simulink model "NeuronalNetwork"  (R2019b)
settings: Solver=VariableStepAuto  StartTime=0.0  StopTime=10.0  RelTol=1e-3
libraries: neural x1006
(part 4 of 11)

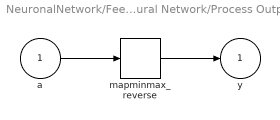
== system NeuronalNetwork/Feed-Forward Neural Network/Process Output 1 ==
  a : Inport  PortDimensions=1001  SampleTime=0.1
      mask Display: e = 0.06;c1 = [120 230 180]/255;c2 = ([120 230 180]+0)/(256+128);c3 = ([120 230 180]+128)/(256+128);patch([0 1 1 0],[0 0 1 1],c1);patch([0 1 1 1-e 1-e 0+e],[0 0 1 1-e 0+e 0+e],c2);patch([0 0 1 1-e 0+e 0+e],[0 1 1 1-e 1-e 0+e],c3);plot([0 1 1 0 0],[0 0 1 1 0]);
  mapminmax_reverse : neural/Processing Functions/mapminmax_reverse  xmin=[1.28539816339744827899949086714;1.20368306698340132854241346649;1.13712353826944823076416923868;1.08663227213241242452568258159;1.04879801985670040309628348041;1.01840689604369138976380781969;0.990200914007079879830541813135;0.959785932234298533316518842184;0.923951810884579005644923199725;0.880690181190778353936821076786;0.82910523056761875615450207988;0.769305868941106085756587162905;0.702287253703623770562103345583;0.629773356468130929286530772515;0.553998001771835668627375071082;0.477432717740583156817990584386;0.402501528649066797616029589335;0.331335469164235618677594175097;0.265607673356772433503891761575;0.206463137107515737334040295536;0.154531156045622314332277369431;0.109993530356310459383806232836;0.0726795004890897489158163580214;0.0421645837339916507158221747886;0.017859386511117698176365209406;-0.0009177424313119231713206658263;-0.0148851418599052279234662421459;-0.0247575410518087804523368333776;-0.0312182369750025681676142141896;-0.0349009375278889616422972608234;-0.0363788753059904115816358682878;-0.0361593048566425795398160403238;-0.034681949339717889346790258287;-0.0323203135455749288040827593704;-0.0293850345279976013501688214546;-0.026128622222722015094875658292;-0.0227510749875170885381248098156;-0.0194059579004072363384025834421;-0.0162066168017704972936776641745;-0.01323227471824351894613691627;-0.0105338220429840728753489997871;-0.00813916833642066434029160859609;-0.00605807183182810026628173361019;-0.00428640265499571643942333665223;-0.00280982765288581310542115332396;-0.00160692915066506809146362755314;-0.000651787741753224840468572409691;8.39286851426477892475219722002e-05;0.000629320082254218463382877679635;0.00101300031231716714842649995632;0.00126218020832500016185917512956;0.00140203514486378095355023631896;0.00145530765965246706647451269134;0.00144209971760712353516797890052;0.00137981388265491153322095385647;0.00128320762461004876306414068665;0.00116452998530110055953878944734;0.00103371466977684837995621336404;0.000898608179116162182273330749638;0.000765215770345728692192199815736;0.000637951762407977778640555399647;0.000519883980299147910320023413533;0.000412964940793953089008538892557;0.00031824474788542760333304171283;0.00023606261194043158622296596505;0.000166215469383906465014599795893;0.000108103400168395807163720934163;6.08524610886519799063387736737e-05;2.34162169208532289070047449631e-05;-5.34230028835631188611002273525e-06;-2.65862022088442081439296077461e-05;-4.14557944757335889362712122441e-05;-5.10329161911559367817425858505e-05;-5.63164827063128490929055924852e-05;-5.82072692902861084764468135866e-05;-5.75001367756681043769476091576e-05;-5.48820875683109677019289041056e-05;-5.09347386144847096077319104079e-05;-4.61399970832799275269331396032e-05;-4.08879171397081897553274498769e-05;-3.54858969220893643442549247879e-05;-3.01685401446361378479353587689e-05;-2.51076545416805896261853991991e-05;-2.04219887447018084341079924293e-05;-1.61864201052371685092372277648e-05;-1.24403991155824628463610545537e-05;-9.19553259175657961867460937766e-06;-6.44224908927785349169181650097e-06;-4.15553778320655725349135056756e-06;-2.29978798182882333719879650036e-06;-8.32782202753131421053595269399e-07;2.91086912351799163033215598478e-07;1.11829527416051354807313179818e-06;1.69427622465038722307149009205e-06;2.06203379837715148698235392843e-06;2.26119730539668068610933450435e-06;2.32743929062701355179113016369e-06;2.29218552361031937175455883149e-06;2.18255324213514291569132944049e-06;2.02146178684901004521346987164e-06;1.8278677282874039293643873838e-06;1.61708423984628104318195251921e-06;1.40115166669096249938190022755e-06;1.18923277936375108412348812481e-06;9.88012053060236007109243955293e-07;8.02083437001456546003590360183e-07;6.34315434400157725518178825075e-07;4.86185998571632601507222330717e-07;3.58082746565454098389104028999e-07;2.49566404431077310633680169105e-07;1.59597261184529452979435990706e-07;8.67258180825558081708905652091e-08;2.92498034681898388953413814306e-08 ...(+32674 chars)]  xmax=[2.00000000000000044408920985006;2.04152251213773938687268127978;2.04743770822412196608297563216;2.04474092985389566123899385275;2.05201540147876348996192064078;2.08123084699771299099779753305;2.14002847333901025095315162616;2.23345756662486705224068828102;2.36503432620028020139102409303;2.53728324397718241201005184848;2.75195877075294292879448221356;3.01012068724373582639941560046;3.31220255873579416672214392747;3.65816820678026033419882878661;4.04779188334038764196520787664;4.48103415237663682546553900465;4.95843958634650316952274806681;5.48147244731911609250118999626;6.05273244640769991775641756249;6.67603631671975428218956949422;7.35638955515603409907043896965;8.09989269105342835075589391636;8.91362727344386129857412015554;9.80555587392072069974346959498;10.7844561957117051065324631054;11.8598972717637991536321351305;13.0422576691496985290541488212;14.3427813376549444512875197688;15.7736651620972718745861129719;17.3481723132318599311929574469;19.0807663529701976301566901384;20.9872622564923076993181894068;23.0849918043823159052863047691;25.3929820358766669130545778899;27.9321465692165489258513844106;30.7254905515174101537922979333;33.798330785307989287957752822;37.1785331959093028331153618637;40.8967702709283784656690841075;44.9868014481570952511901850812;49.485779684486061569259618409;54.4345876406889956911072658841;59.878207097440551365252758842;65.8661254044489510306448210031;72.4527829791836097683699335903;79.6980661306850350911190616898;87.6678497985661948632696294226;96.4345951746557830119854770601;106.078007618962104174897831399;116.685760795105608167432365008;128.354293534616601846209960058;141.189686596049426725585362874;155.308627215846740909910295159;170.839470156436959769052919;187.923404847583896071228082292;206.715739195378546355641447008;227.387311706783407316834200174;250.126044755114776307891588658;275.138653103523267873242730275;302.652523221087051297217840329;332.917780482648197448725113645;366.209563053505860352743184194;402.830523139516571973217651248;443.113578349547537982289213687;487.424938189776071340020280331;536.167433209015143802389502525;589.784177064038431126391515136;648.762594798973736942571122199;713.638853960809569798584561795;785.002738834249839783296920359;863.503012106822438909148331732;949.853312705906660085020121187;1044.8386434234166699752677232;1149.32250730554164874774869531;1264.25475768286923994310200214;1390.68023320400084230641368777;1529.74825637233561792527325451;1682.7230819359069755591917783;1850.99539011534693599969614297;2036.09492915372288734943140298;2239.70442212048283181502483785;2463.67486439503272777074016631;2710.04235089806707037496380508;2981.0465860455942674889229238;3279.15124469807597051840275526;3607.06636920432902115862816572;3967.77300614976275028311647475;4364.55030677947524964110925794;4801.00533746372093446552753448;5281.10587121003482025116682053;5809.21645832666126807453110814;6390.13810415244461182737722993;7029.1519145597694659954868257;7732.06710600789028831059113145;8505.27381660162609477993100882;9355.80119825595829752273857594;10291.3813180771048791939392686;11320.5194498817272688029333949;12452.5713948680277098901569843;13697.8285343539500900078564882;15067.6113877892130403779447079;16574.3725265685134218074381351;18231.8097792260414280463010073;20054.9907571494622970931231976;22060.4898328652197960764169693;24266.538816152482468169182539;26693.1926977683360746596008539;29362.511967545629886444658041;32298.7631643005042860750108957;35528.6394807307369774207472801;39081.503428803880524355918169;42989.6537716842649388127028942;47288.6191488526310422457754612;52017.4810637378031970001757145;57219.2291701114736497402191162;62941.1520871225220616906881332;69235.2672958346811356022953987;76158.7940254180866759270429611;83774.6734279598458670079708099;92152.1407707557955291122198105;101367.354847831345978192985058;111504.090332614461658522486687;122654.499365875904913991689682;134919.949302463501226156949997;148411.94423270988045260310173 ...(+25334 chars)]  ymin=-1  ymax=1
      settings: SourceProductName=Deep Learning Toolbox
  y : Outport  PortDimensions=1001  SampleTime=0.1
      mask Display: e = 0.06;c1 = [120 230 180]/255;c2 = ([120 230 180]+0)/(256+128);c3 = ([120 230 180]+128)/(256+128);patch([0 1 1 0],[0 0 1 1],c1);patch([0 1 1 1-e 1-e 0+e],[0 0 1 1-e 0+e 0+e],c2);patch([0 0 1 1-e 0+e 0+e],[0 1 1 1-e 1-e 0+e],c3);plot([0 1 1 0 0],[0 0 1 1 0]);
  wires:
  a/1 -> mapminmax_reverse/1
  mapminmax_reverse/1 -> y/1
